simulink model "flywheel_speed_ctrl_with_load_observer_ccode"  (R2021b)
settings: Solver=ode23tb  StartTime=0.0  StopTime=simulation_length  MaxStep=ts
undefined symbols (not defined in the file): A, Aed, B, Bed, C, Ce, E, ki, kp, Led, Tc, ts
settings Model: SimulationMode=accelerator  Creator=dbagn  LastModifiedBy=dbagn
settings SolverCC: AlgebraicLoopSolver=TrustRegion
settings DataIOCC: SaveTime=off  ReturnWorkspaceOutputs=off
settings DebuggingCC: SFMachineParentedDataDiag=warning
settings SFSimCC: SimCustomHeaderCode="#include \"sfbctrl.h\""  SimUserSources=src/sfbctrl.c  SimUserIncludeDirs=include

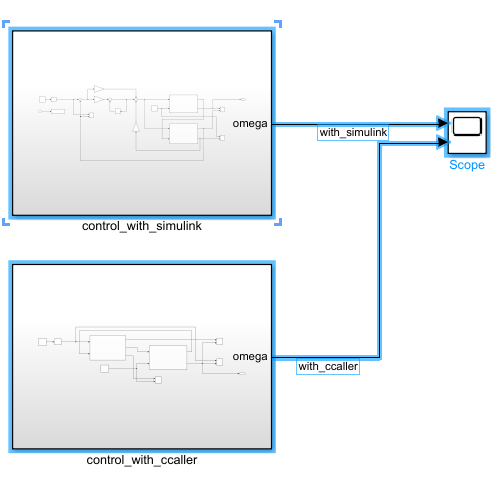
[thumbnail: Simulink's stored preview of the top-level diagram]
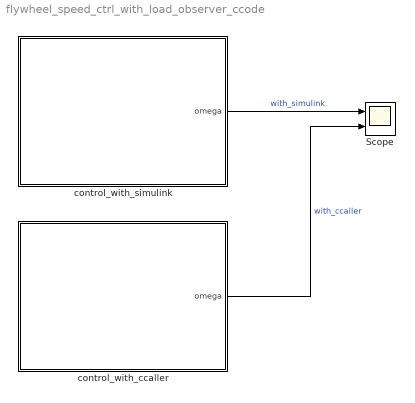
== system flywheel_speed_ctrl_with_load_observer_ccode ==
  Scope : Scope  NumInputPorts=2
  control_with_ccaller : Subsystem
  control_with_simulink : Subsystem
  wires:
  control_with_simulink/1(omega) -> Scope/1  "with_simulink"
  control_with_ccaller/1(omega) -> Scope/2  "with_ccaller"

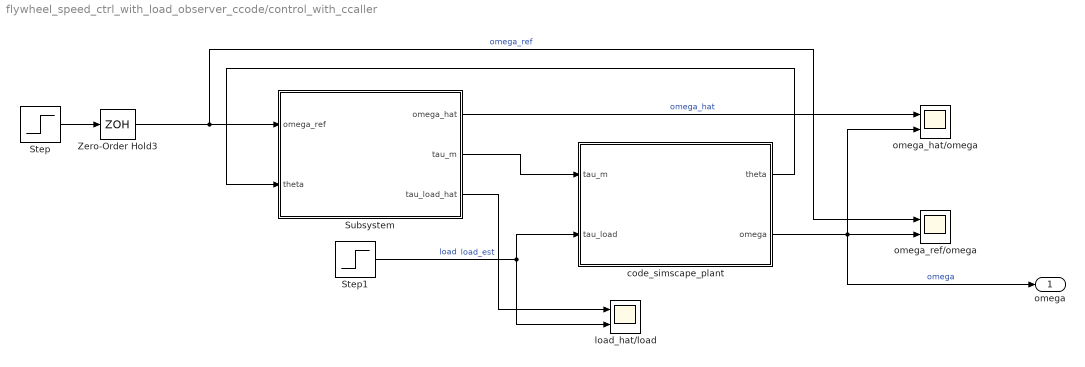
== system flywheel_speed_ctrl_with_load_observer_ccode/control_with_ccaller ==
  Step : Step  Time=0.2  SampleTime=0
  Step1 : Step  After=25  SampleTime=0
  Subsystem : Subsystem
  Zero-Order Hold3 : ZeroOrderHold  SampleTime=ts
  "code_simscape_plant " : Subsystem
  load_hat/load : Scope  NumInputPorts=2
  omega_hat/omega : Scope  NumInputPorts=2
  omega_ref/omega : Scope  NumInputPorts=2
  omega : Outport
  wires:
  Step/1 -> Zero-Order Hold3/1
  Zero-Order Hold3/1 -> omega_ref/omega/1, Subsystem/1(omega_ref)  "omega_ref"
  Step1/1 -> "code_simscape_plant "/2(tau_load), load_hat/load/2  "load"
  "code_simscape_plant "/1(theta) -> Subsystem/2(theta)
  Subsystem/1(omega_hat) -> omega_hat/omega/1  "omega_hat"
  Subsystem/3(tau_load_hat) -> load_hat/load/1  "load_est"
  Subsystem/2("tau_m ") -> "code_simscape_plant "/1(tau_m)
  "code_simscape_plant "/2(omega) -> omega_hat/omega/2, omega/1, omega_ref/omega/2  "omega"

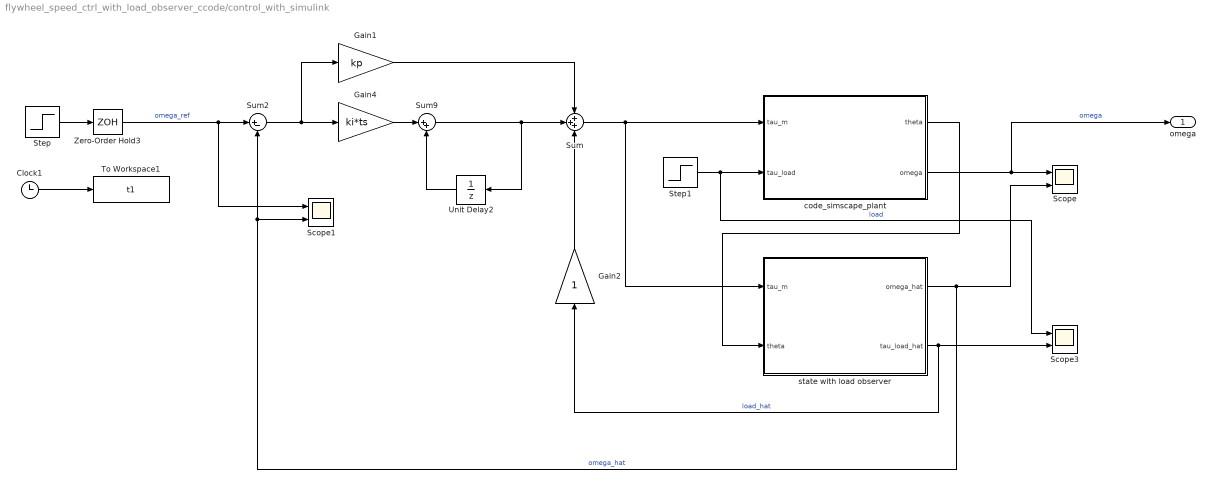
== system flywheel_speed_ctrl_with_load_observer_ccode/control_with_simulink ==
  Clock1 : Clock
  Gain1 : Gain  Gain=kp
  Gain2 : Gain
  Gain4 : Gain  Gain=ki*ts
  Scope : Scope  NumInputPorts=2
  Scope1 : Scope  NumInputPorts=2
  Scope3 : Scope  NumInputPorts=2
  Step : Step  Time=0.2  SampleTime=0
  Step1 : Step  After=25  SampleTime=0
  Sum : Sum  Inputs=+++
  Sum2 : Sum  Inputs=|+-
  Sum9 : Sum  Inputs=|++
  To Workspace1 : ToWorkspace  VariableName=t1  SampleTime=Tc
      settings: MaxDataPoints=Nc
  Unit Delay2 : UnitDelay  SampleTime=ts  HasFrameUpgradeWarning=on
  Zero-Order Hold3 : ZeroOrderHold  SampleTime=ts
  "code_simscape_plant " : Subsystem
  state with load observer : Subsystem
  omega : Outport
  wires:
  Gain2/1 -> Sum/3
  state with load observer/1(omega_hat) -> Scope/2, Scope1/2, Sum2/2  "omega_hat"
  state with load observer/2(tau_load_hat) -> Gain2/1, Scope3/2  "load_hat"
  Step1/1 -> "code_simscape_plant "/2(tau_load), Scope3/1  "load"
  "code_simscape_plant "/2(omega) -> omega/1, Scope/1  "omega"
  Sum/1 -> state with load observer/1(tau_m), "code_simscape_plant "/1(tau_m)
  "code_simscape_plant "/1(theta) -> state with load observer/2(theta)
  Zero-Order Hold3/1 -> Scope1/1, Sum2/1  "omega_ref"
  Sum2/1 -> Gain1/1, Gain4/1
  Sum9/1 -> Unit Delay2/1, Sum/2
  Unit Delay2/1 -> Sum9/2
  Gain1/1 -> Sum/1
  Step/1 -> Zero-Order Hold3/1
  Gain4/1 -> Sum9/1
  Clock1/1 -> To Workspace1/1

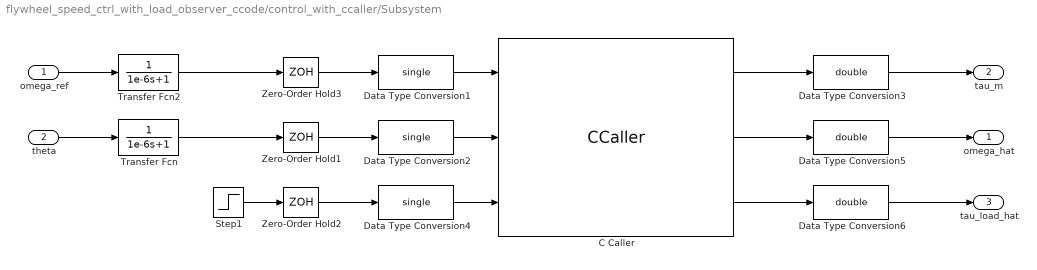
== system flywheel_speed_ctrl_with_load_observer_ccode/control_with_ccaller/Subsystem ==
  omega_ref : Inport
  theta : Inport  Port=2
  C Caller : CCaller  FunctionName=ctrlSimulink  PortSpecificationStruct="%)30     .    R H   8    (     @         %    \"     8    !     0         %  0 \"0    $    _    07)G3F%M90  4&]R=$YA;64 4V-O<&4     26YD97@     5'EP90      4VEZ90      27-';&]B86P   X   !     !@    @    $          4    (     0    D    !         !     )    ;VUE9V%?<F5F          X   !     !@    @    $          4    (     0    D    !         !     )    ;VUE9V%?<F5F          X    X    !@    @    $     ...(+3337 chars)"
  Data Type Conversion1 : DataTypeConversion  OutDataTypeStr=single
  Data Type Conversion2 : DataTypeConversion  OutDataTypeStr=single
  Data Type Conversion3 : DataTypeConversion  OutDataTypeStr=double
  Data Type Conversion4 : DataTypeConversion  OutDataTypeStr=single
  Data Type Conversion5 : DataTypeConversion  OutDataTypeStr=double
  Data Type Conversion6 : DataTypeConversion  OutDataTypeStr=double
  Step1 : Step  Time=0.1  Before=1  After=0  SampleTime=0
  Transfer Fcn : TransferFcn  Denominator=[1e-6 1]
  Transfer Fcn2 : TransferFcn  Denominator=[1e-6 1]
  Zero-Order Hold1 : ZeroOrderHold  SampleTime=ts
  Zero-Order Hold2 : ZeroOrderHold  SampleTime=ts
  Zero-Order Hold3 : ZeroOrderHold  SampleTime=ts
  omega_hat : Outport
  "tau_m " : Outport  Port=2
  tau_load_hat : Outport  Port=3
  wires:
  Data Type Conversion1/1 -> C Caller/1
  Step1/1 -> Zero-Order Hold2/1
  Zero-Order Hold2/1 -> Data Type Conversion4/1
  Data Type Conversion3/1 -> "tau_m "/1
  Zero-Order Hold3/1 -> Data Type Conversion1/1
  Zero-Order Hold1/1 -> Data Type Conversion2/1
  theta/1 -> Transfer Fcn/1
  Data Type Conversion5/1 -> omega_hat/1
  Transfer Fcn/1 -> Zero-Order Hold1/1
  omega_ref/1 -> Transfer Fcn2/1
  Transfer Fcn2/1 -> Zero-Order Hold3/1
  Data Type Conversion2/1 -> C Caller/2
  Data Type Conversion4/1 -> C Caller/3
  C Caller/2 -> Data Type Conversion5/1
  C Caller/1 -> Data Type Conversion3/1
  Data Type Conversion6/1 -> tau_load_hat/1
  C Caller/3 -> Data Type Conversion6/1

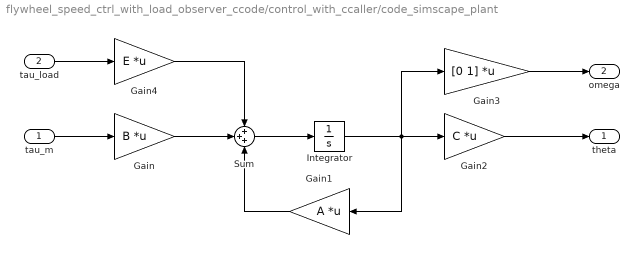
== system flywheel_speed_ctrl_with_load_observer_ccode/control_with_ccaller/code_simscape_plant  ==
  tau_m : Inport
  tau_load : Inport  Port=2
  Gain : Gain  Gain=B  Multiplication=Matrix(K*u)
  Gain1 : Gain  Gain=A  Multiplication=Matrix(K*u)
  Gain2 : Gain  Gain=C  Multiplication=Matrix(K*u)
  Gain3 : Gain  Gain=[0 1]  Multiplication=Matrix(K*u)
  Gain4 : Gain  Gain=E  Multiplication=Matrix(K*u)
  Integrator : Integrator
  Sum : Sum  Inputs=+++
  theta : Outport
  omega : Outport  Port=2
  wires:
  Gain4/1 -> Sum/1
  Gain1/1 -> Sum/3
  Gain/1 -> Sum/2
  tau_load/1 -> Gain4/1
  Gain3/1 -> omega/1
  tau_m/1 -> Gain/1
  Gain2/1 -> theta/1
  Integrator/1 -> Gain1/1, Gain2/1, Gain3/1
  Sum/1 -> Integrator/1

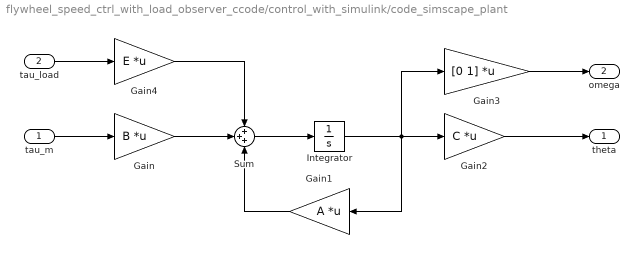
== system flywheel_speed_ctrl_with_load_observer_ccode/control_with_simulink/code_simscape_plant  ==
  tau_m : Inport
  tau_load : Inport  Port=2
  Gain : Gain  Gain=B  Multiplication=Matrix(K*u)
  Gain1 : Gain  Gain=A  Multiplication=Matrix(K*u)
  Gain2 : Gain  Gain=C  Multiplication=Matrix(K*u)
  Gain3 : Gain  Gain=[0 1]  Multiplication=Matrix(K*u)
  Gain4 : Gain  Gain=E  Multiplication=Matrix(K*u)
  Integrator : Integrator
  Sum : Sum  Inputs=+++
  theta : Outport
  omega : Outport  Port=2
  wires:
  Sum/1 -> Integrator/1
  Integrator/1 -> Gain3/1, Gain2/1, Gain1/1
  Gain2/1 -> theta/1
  tau_m/1 -> Gain/1
  Gain3/1 -> omega/1
  tau_load/1 -> Gain4/1
  Gain/1 -> Sum/2
  Gain1/1 -> Sum/3
  Gain4/1 -> Sum/1

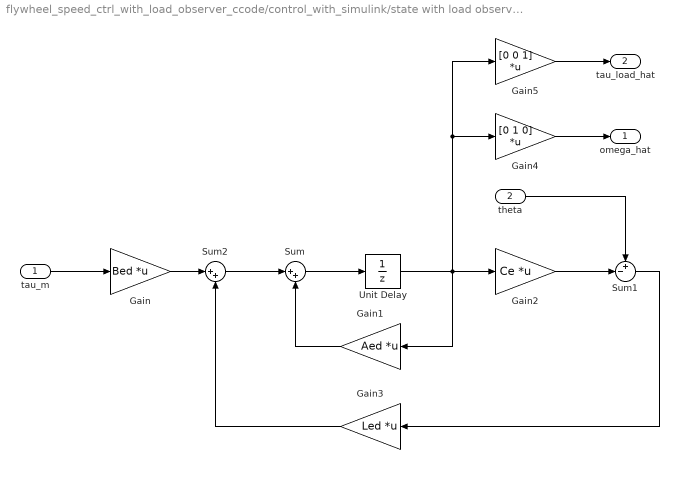
== system flywheel_speed_ctrl_with_load_observer_ccode/control_with_simulink/state with load observer ==
  tau_m : Inport
  theta : Inport  Port=2
  Gain : Gain  Gain=Bed  Multiplication=Matrix(K*u)
  Gain1 : Gain  Gain=Aed  Multiplication=Matrix(K*u)
  Gain2 : Gain  Gain=Ce  Multiplication=Matrix(K*u)
  Gain3 : Gain  Gain=Led  Multiplication=Matrix(K*u)
  Gain4 : Gain  Gain=[0 1 0]  Multiplication=Matrix(K*u)
  Gain5 : Gain  Gain=[0 0 1]  Multiplication=Matrix(K*u)
  Sum : Sum  Inputs=|++
  Sum1 : Sum  Inputs=+-|
  Sum2 : Sum  Inputs=|++
  Unit Delay : UnitDelay  SampleTime=ts  HasFrameUpgradeWarning=on
  omega_hat : Outport
  tau_load_hat : Outport  Port=2
  wires:
  Sum/1 -> Unit Delay/1
  tau_m/1 -> Gain/1
  Gain1/1 -> Sum/2
  Gain2/1 -> Sum1/2
  theta/1 -> Sum1/1
  Gain/1 -> Sum2/1
  Sum2/1 -> Sum/1
  Sum1/1 -> Gain3/1
  Gain3/1 -> Sum2/2
  Unit Delay/1 -> Gain5/1, Gain4/1, Gain2/1, Gain1/1
  Gain4/1 -> omega_hat/1
  Gain5/1 -> tau_load_hat/1
